simulink model "feedbackLin_Sim_Model"  (R2021a)
settings: Solver=ode1  StartTime=0.0  StopTime=200  FixedStep=0.005  RelTol=1e-3
values from neighbouring files (symbols this model uses):
  g = 9.31    [Metrics_Info.m]    (also in initEnv.m)
undefined symbols (not defined in the file or in its folder): Controller, DiscIntNeverNeededParam, Earth, init, rho, Vehicle, WGS84
libraries: shared6dof x1, aerolibasang x1, dynamicsLibrary x1, aerolibtransform2 x1
settings Model: Creator=laberobotica  LastModifiedBy=laberobotica

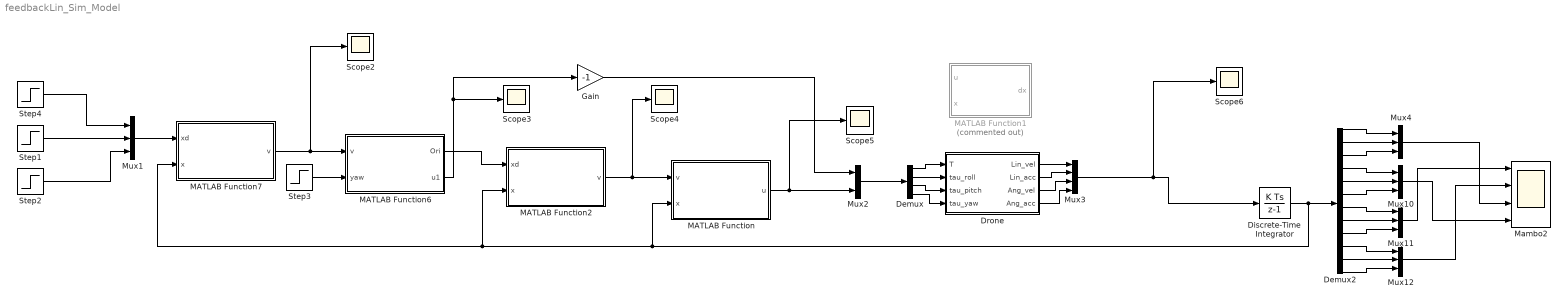
== system feedbackLin_Sim_Model ==
  Demux : Demux
  Demux2 : Demux  Outputs=12
  Discrete-Time Integrator : DiscreteIntegrator  SampleTime=0.005  ICPrevOutput=DiscIntNeverNeededParam  ICPrevScaledInput=DiscIntNeverNeededParam
  Drone : Subsystem
  Gain : Gain  Gain=-1
  MATLAB Function : MATLAB Function  TreatAsAtomicUnit=on
  MATLAB Function1 : MATLAB Function  Commented=on  TreatAsAtomicUnit=on
  MATLAB Function2 : MATLAB Function  TreatAsAtomicUnit=on
  MATLAB Function6 : MATLAB Function  TreatAsAtomicUnit=on
  MATLAB Function7 : MATLAB Function  TreatAsAtomicUnit=on
  Mambo2 : Scope  NumInputPorts=4
  Mux{1,4,10..12} (5 alike) : Mux  Inputs=3
  Mux2 : Mux  Inputs=2
  Mux3 : Mux
  Scope{2..6} (5 alike) : Scope
  Step1 : Step  Time=30  SampleTime=0
  Step2 : Step  Time=5  SampleTime=0.005
  Step3 : Step  Time=100  SampleTime=0.005
  Step4 : Step  Time=50  SampleTime=0
  wires:
  MATLAB Function2/1(v) -> Scope4/1, MATLAB Function/1(v)
  Mux1/1 -> MATLAB Function7/1(xd)
  Step2/1 -> Mux1/3
  MATLAB Function7/1(v) -> Scope2/1, MATLAB Function6/1(v)
  Demux2/7 -> Mux11/1
  Demux2/9 -> Mux11/3
  Demux2/2 -> Mux4/2
  Demux2/10 -> Mux12/1
  Mux11/1 -> Mambo2/1
  Mux4/1 -> Mambo2/3
  Demux2/8 -> Mux11/2
  Discrete-Time Integrator/1 -> MATLAB Function2/2(x), MATLAB Function7/2(x), MATLAB Function/2(x), Demux2/1
  Mux10/1 -> Mambo2/4
  Mux12/1 -> Mambo2/2
  Demux2/3 -> Mux4/3
  Demux2/11 -> Mux12/2
  Demux2/6 -> Mux10/3
  Demux2/12 -> Mux12/3
  Demux2/4 -> Mux10/1
  Demux2/5 -> Mux10/2
  Demux2/1 -> Mux4/1
  MATLAB Function6/2(u1) -> Gain/1, Scope3/1
  MATLAB Function6/1(Ori) -> MATLAB Function2/1(xd)
  Step4/1 -> Mux1/1
  Step1/1 -> Mux1/2
  Step3/1 -> MATLAB Function6/2(yaw)
  Drone/1(Lin_vel) -> Mux3/1
  Drone/2(Lin_acc) -> Mux3/2
  Drone/3(Ang_vel) -> Mux3/3
  Drone/4(Ang_acc) -> Mux3/4
  Demux/1 -> Drone/1(T)
  Demux/2 -> Drone/2(tau_roll)
  Demux/3 -> Drone/3(tau_pitch)
  Demux/4 -> Drone/4(tau_yaw)
  Mux3/1 -> Scope6/1, Discrete-Time Integrator/1
  Mux2/1 -> Demux/1
  Gain/1 -> Mux2/1
  MATLAB Function/1(u) -> Mux2/2, Scope5/1

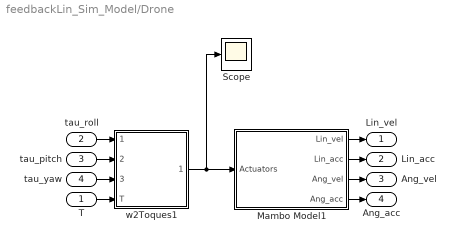
== system feedbackLin_Sim_Model/Drone ==
  T : Inport
  tau_roll : Inport  Port=2
  tau_pitch : Inport  Port=3
  tau_yaw : Inport  Port=4
  Mambo Model1 : Subsystem
  Scope : Scope
  w2Toques1 : Subsystem
  Lin_vel : Outport
  Lin_acc : Outport  Port=2
  Ang_vel : Outport  Port=3
  Ang_acc : Outport  Port=4
  wires:
  tau_yaw/1 -> w2Toques1/3(tau_yaw)
  tau_pitch/1 -> w2Toques1/2(tau_pitch)
  Mambo Model1/1(Lin_vel) -> Lin_vel/1
  Mambo Model1/4(Ang_acc) -> Ang_acc/1
  w2Toques1/1(Motors) -> Scope/1, Mambo Model1/1(Actuators)
  T/1 -> w2Toques1/4(T)
  Mambo Model1/3(Ang_vel) -> Ang_vel/1
  tau_roll/1 -> w2Toques1/1(tau_roll)
  Mambo Model1/2(Lin_acc) -> Lin_acc/1

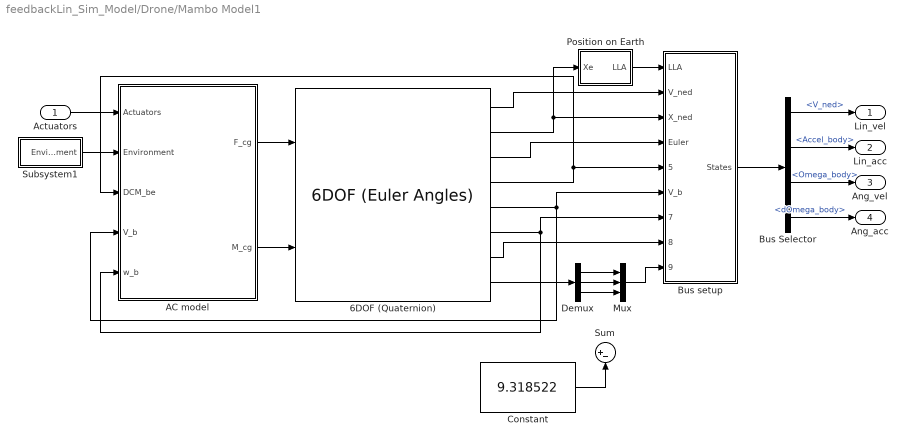
== system feedbackLin_Sim_Model/Drone/Mambo Model1 ==
  Actuators : Inport
  6DOF (Quaternion) : shared6dof/6DOF (Euler Angles)  units=Metric (MKS)  mtype=Fixed  rep=Euler Angles  xme_0=[0 0 0]  Vm_0=init.vb  eul_0=init.euler  pm_0=init.angRates  mass_0=Vehicle.Airframe.mass  mass_e=0.5  mass_f=2.0  inertia=Vehicle.Airframe.inertia  inertia_e=eye(3)  inertia_f=2*eye(3)  k_quat=Vehicle.SixDOF.quatGain  vre_flag=on  abi_flag=off  aMode=aMode  xme_statename=''  Vm_statename=''  eul_statename=''  quat_statename=''  pm_statename=''  mass_statename=''
      settings: SourceProductBaseCode=AE,PW,DR,MT,UV,VE
  AC model : Subsystem
  Bus Selector : BusSelector  OutputSignals=V_ned,Accel_body,Omega_body,dOmega_body
  Bus setup : Subsystem
  Constant : Constant  Value=9.318522
  Demux : Demux  Outputs=3
  Mux : Mux  Inputs=3
  Position on Earth : Subsystem  Priority=1  TreatAsAtomicUnit=on
  Subsystem1 : Subsystem
  Sum : Sum  Inputs=|+-
  Lin_vel : Outport
  Lin_acc : Outport  Port=2
  Ang_vel : Outport  Port=3
  Ang_acc : Outport  Port=4
  wires:
  Position on Earth/1(LLA) -> Bus setup/1(LLA)
  6DOF (Quaternion)/5 -> Bus setup/6(V_b), AC model/4(V_b)
  6DOF (Quaternion)/7 -> Bus setup/8(dOmega_b)
  Subsystem1/1(Environment) -> AC model/2(Environment)
  6DOF (Quaternion)/1 -> Bus setup/2(V_ned)
  Bus setup/1(States) -> Bus Selector/1
  AC model/1(F_cg) -> 6DOF (Quaternion)/1
  6DOF (Quaternion)/6 -> Bus setup/7(Omega_b), AC model/5(w_b)
  6DOF (Quaternion)/2 -> Position on Earth/1(Xe), Bus setup/3(X_ned)
  6DOF (Quaternion)/3 -> Bus setup/4(Euler)
  Actuators/1 -> AC model/1(Actuators)
  AC model/2(M_cg) -> 6DOF (Quaternion)/2
  6DOF (Quaternion)/4 -> AC model/3(DCM_be), Bus setup/5(DCM_be)
  Bus Selector/1 -> Lin_vel/1  "<V_ned>"
  Bus Selector/2 -> Lin_acc/1  "<Accel_body>"
  Bus Selector/3 -> Ang_vel/1  "<Omega_body>"
  Bus Selector/4 -> Ang_acc/1  "<dOmega_body>"
  Constant/1 -> Sum/2
  6DOF (Quaternion)/8 -> Demux/1
  Mux/1 -> Bus setup/9(Accel_b)
  Demux/1 -> Mux/1
  Demux/2 -> Mux/2
  Demux/3 -> Mux/3

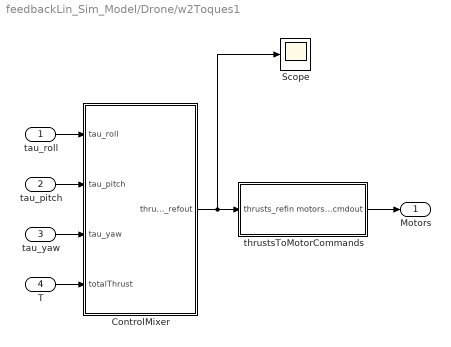
== system feedbackLin_Sim_Model/Drone/w2Toques1 ==
  tau_roll : Inport
  tau_pitch : Inport  Port=2
  tau_yaw : Inport  Port=3
  T : Inport  Port=4
  ControlMixer : Subsystem
  Scope : Scope
  thrustsToMotorCommands : Subsystem
  Motors : Outport  VectorParamsAs1DForOutWhenUnconnected=off
  wires:
  ControlMixer/1(thrusts_refout) -> Scope/1, thrustsToMotorCommands/1(thrusts_refin)
  thrustsToMotorCommands/1(motors_cmdout) -> Motors/1
  tau_roll/1 -> ControlMixer/1(tau_roll)
  tau_pitch/1 -> ControlMixer/2(tau_pitch)
  tau_yaw/1 -> ControlMixer/3(tau_yaw)
  T/1 -> ControlMixer/4(totalThrust)

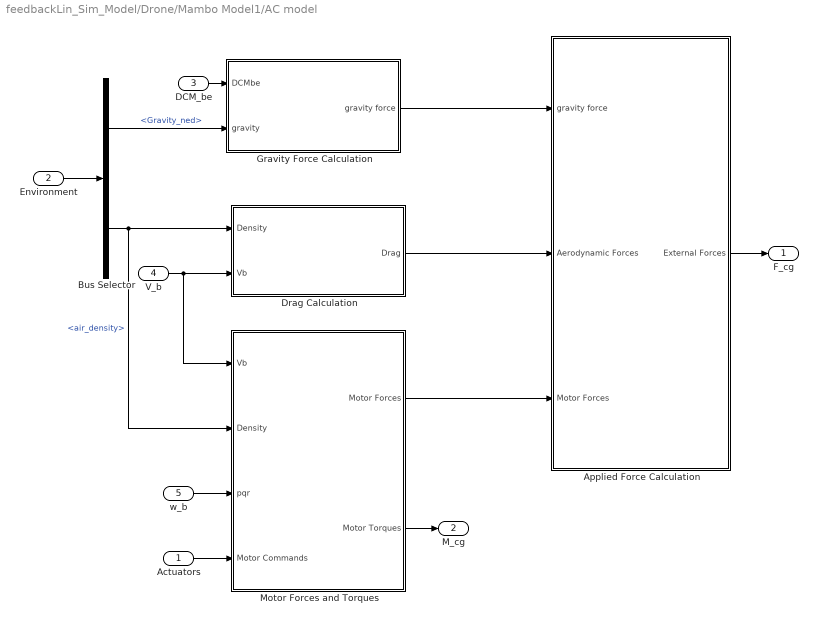
== system feedbackLin_Sim_Model/Drone/Mambo Model1/AC model ==
  Actuators : Inport
  Environment : Inport  Port=2
  DCM_be : Inport  Port=3
  V_b : Inport  Port=4  Unit=m/s
  w_b : Inport  Port=5  Unit=rad/s
  Applied Force Calculation : Subsystem
  Bus Selector : BusSelector  OutputSignals=Gravity_ned,AtmosphereBus.air_density
  Drag Calculation : Subsystem
  Gravity Force Calculation : Subsystem
  Motor Forces and Torques : Subsystem
  F_cg : Outport  Unit=N  VectorParamsAs1DForOutWhenUnconnected=off
  M_cg : Outport  Port=2  Unit=N*m  VectorParamsAs1DForOutWhenUnconnected=off
  wires:
  Bus Selector/1 -> Gravity Force Calculation/2(gravity)  "<Gravity_ned>"
  Gravity Force Calculation/1(gravity force) -> Applied Force Calculation/1(gravity force)
  Environment/1 -> Bus Selector/1
  Bus Selector/2 -> Motor Forces and Torques/2(Density), Drag Calculation/1(Density)  "<air_density>"
  DCM_be/1 -> Gravity Force Calculation/1(DCMbe)
  V_b/1 -> Motor Forces and Torques/1(Vb), Drag Calculation/2(Vb)
  Drag Calculation/1(Drag) -> Applied Force Calculation/2(Aerodynamic Forces)
  Actuators/1 -> Motor Forces and Torques/4(Motor Commands)
  w_b/1 -> Motor Forces and Torques/3(pqr)
  Motor Forces and Torques/2(Motor Torques) -> M_cg/1
  Applied Force Calculation/1(External Forces) -> F_cg/1
  Motor Forces and Torques/1(Motor Forces) -> Applied Force Calculation/3(Motor Forces)

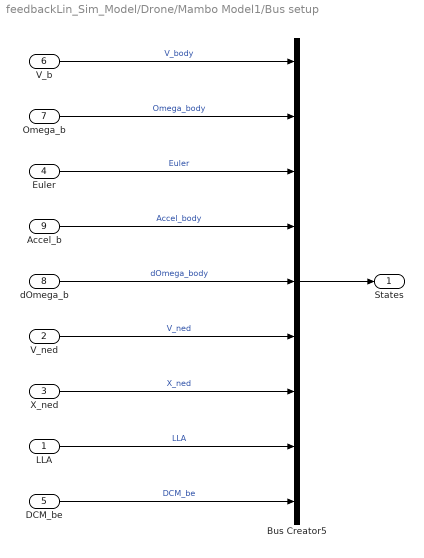
== system feedbackLin_Sim_Model/Drone/Mambo Model1/Bus setup ==
  LLA : Inport  PortDimensions=3
  V_ned : Inport  Port=2  Unit=m/second  PortDimensions=3
  X_ned : Inport  Port=3  Unit=m  PortDimensions=3
  Euler : Inport  Port=4  Unit=rad  PortDimensions=3
  DCM_be : Inport  Port=5  PortDimensions=[3 3]
  V_b : Inport  Port=6  Unit=m/s  PortDimensions=3
  Omega_b : Inport  Port=7  Unit=rad/s  PortDimensions=3
  dOmega_b : Inport  Port=8  Unit=rad/s^2  PortDimensions=3
  Accel_b : Inport  Port=9  Unit=m/s^2  PortDimensions=3
  Bus Creator5 : BusCreator  Inputs=9  OutDataTypeStr=Bus: StatesBus  NonVirtualBus=on
  States : Outport  VectorParamsAs1DForOutWhenUnconnected=off
  wires:
  Bus Creator5/1 -> States/1
  V_b/1 -> Bus Creator5/1  "V_body"
  Omega_b/1 -> Bus Creator5/2  "Omega_body"
  Euler/1 -> Bus Creator5/3  "Euler"
  X_ned/1 -> Bus Creator5/7  "X_ned"
  Accel_b/1 -> Bus Creator5/4  "Accel_body"
  LLA/1 -> Bus Creator5/8  "LLA"
  dOmega_b/1 -> Bus Creator5/5  "dOmega_body"
  DCM_be/1 -> Bus Creator5/9  "DCM_be"
  V_ned/1 -> Bus Creator5/6  "V_ned"

== system feedbackLin_Sim_Model/Drone/Mambo Model1/Position on Earth ==
  Xe : Inport  Unit=m
  Flat Earth to LLA : aerolibtransform2/Flat Earth to LLA  units=Metric (MKS)  ptype=Earth (WGS84)  F=1/298.257223563  R=6378137  refPosPort=off  LL0=init.posLLA(1:2)  psi=Vehicle.PositionOnEarth.FlatEarthToLLA.xAxis
  Mux : Mux  Inputs=2
  href : Constant  Value=Vehicle.PositionOnEarth.href
  LLA : Outport  VectorParamsAs1DForOutWhenUnconnected=off
  wires:
  Mux/1 -> LLA/1
  Xe/1 -> Flat Earth to LLA/1
  Flat Earth to LLA/1 -> Mux/1
  Flat Earth to LLA/2 -> Mux/2
  href/1 -> Flat Earth to LLA/2

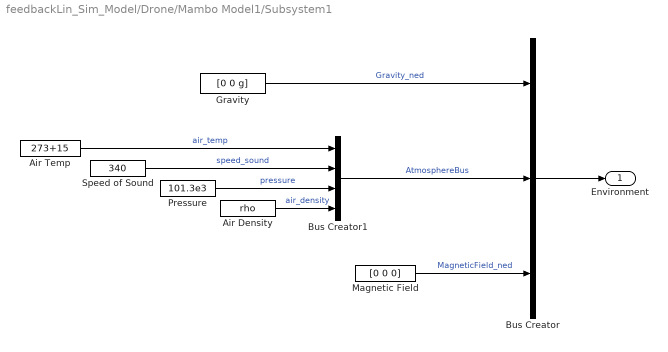
== system feedbackLin_Sim_Model/Drone/Mambo Model1/Subsystem1 ==
  Air Density : Constant  Value=rho
  Air Temp : Constant  Value=273+15
  Bus Creator : BusCreator  Inputs=3  OutDataTypeStr=Bus: EnvironmentBus  NonVirtualBus=on
  Bus Creator1 : BusCreator  Inputs=4  OutDataTypeStr=Bus: AtmosphereBus  NonVirtualBus=on
  Gravity : Constant  Value=[0 0 g]
  Magnetic Field : Constant  Value=[0 0 0]
  Pressure : Constant  Value=101.3e3
  Speed of Sound : Constant  Value=340
  Environment : Outport  VectorParamsAs1DForOutWhenUnconnected=off
  wires:
  Bus Creator1/1 -> Bus Creator/2  "AtmosphereBus"
  Gravity/1 -> Bus Creator/1  "Gravity_ned"
  Air Density/1 -> Bus Creator1/4  "air_density"
  Air Temp/1 -> Bus Creator1/1  "air_temp"
  Speed of Sound/1 -> Bus Creator1/2  "speed_sound"
  Magnetic Field/1 -> Bus Creator/3  "MagneticField_ned"
  Bus Creator/1 -> Environment/1
  Pressure/1 -> Bus Creator1/3  "pressure"

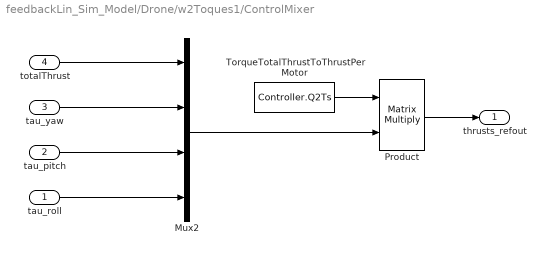
== system feedbackLin_Sim_Model/Drone/w2Toques1/ControlMixer ==
  tau_roll : Inport
  tau_pitch : Inport  Port=2
  tau_yaw : Inport  Port=3
  totalThrust : Inport  Port=4
  Mux2 : Mux
  Product : Product  Multiplication=Matrix(*)  RndMeth=Zero
  TorqueTotalThrustToThrustPerMotor : Constant  Value=Controller.Q2Ts  OutDataTypeStr=single
  thrusts_refout : Outport  VectorParamsAs1DForOutWhenUnconnected=off
  wires:
  Product/1 -> thrusts_refout/1
  tau_roll/1 -> Mux2/4
  tau_yaw/1 -> Mux2/2
  totalThrust/1 -> Mux2/1
  TorqueTotalThrustToThrustPerMotor/1 -> Product/1
  Mux2/1 -> Product/2
  tau_pitch/1 -> Mux2/3

== system feedbackLin_Sim_Model/Drone/w2Toques1/thrustsToMotorCommands ==
  thrusts_refin : Inport
  MotorDirections : Gain  Gain=[1 -1 1 -1]
  Saturation5 : Saturate  UpperLimit=Vehicle.Motor.maxLimit  LowerLimit=Vehicle.Motor.minLimit
  ThrustToMotorCommand : Gain  Gain=-Vehicle.Motor.thrustToMotorCommand
  motors_cmdout : Outport  VectorParamsAs1DForOutWhenUnconnected=off
  wires:
  Saturation5/1 -> MotorDirections/1
  MotorDirections/1 -> motors_cmdout/1
  ThrustToMotorCommand/1 -> Saturation5/1
  thrusts_refin/1 -> ThrustToMotorCommand/1

== system feedbackLin_Sim_Model/Drone/Mambo Model1/AC model/Applied Force Calculation ==
  gravity force : Inport  Unit=N
  Aerodynamic Forces : Inport  Port=2  Unit=N
  Motor Forces : Inport  Port=3  Unit=N
  Add1 : Sum  Inputs=+++
  Signal Specification : SignalSpecification  Dimensions=3
  External Forces : Outport  Unit=N  VectorParamsAs1DForOutWhenUnconnected=off
  wires:
  Add1/1 -> Signal Specification/1
  Motor Forces/1 -> Add1/3  "Motor Thrust"
  Aerodynamic Forces/1 -> Add1/2
  gravity force/1 -> Add1/1
  Signal Specification/1 -> External Forces/1

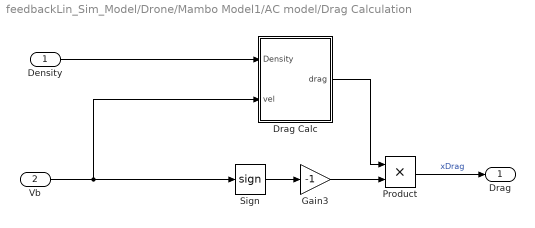
== system feedbackLin_Sim_Model/Drone/Mambo Model1/AC model/Drag Calculation ==
  Density : Inport  Unit=kg/m^3
  Vb : Inport  Port=2  Unit=m/second
  Drag Calc : Subsystem
  Gain3 : Gain  Gain=-1
  Product : Product  RndMeth=Zero
  Sign : Signum  ZeroCross=off
  Drag : Outport  Unit=N  VectorParamsAs1DForOutWhenUnconnected=off
  wires:
  Density/1 -> Drag Calc/1(Density)
  Sign/1 -> Gain3/1
  Drag Calc/1(drag) -> Product/1
  Gain3/1 -> Product/2
  Product/1 -> Drag/1  "xDrag"
  Vb/1 -> Sign/1, Drag Calc/2(vel)

== system feedbackLin_Sim_Model/Drone/Mambo Model1/AC model/Gravity Force Calculation ==
  DCMbe : Inport
  gravity : Inport  Port=2  Unit=m/s^2
  Gain1 : Gain  Gain=Vehicle.Airframe.mass
  Product : Product  Multiplication=Matrix(*)
  gravity force : Outport  Unit=N  VectorParamsAs1DForOutWhenUnconnected=off
  wires:
  gravity/1 -> Gain1/1
  Gain1/1 -> Product/2  "gravity force NED"
  Product/1 -> gravity force/1
  DCMbe/1 -> Product/1

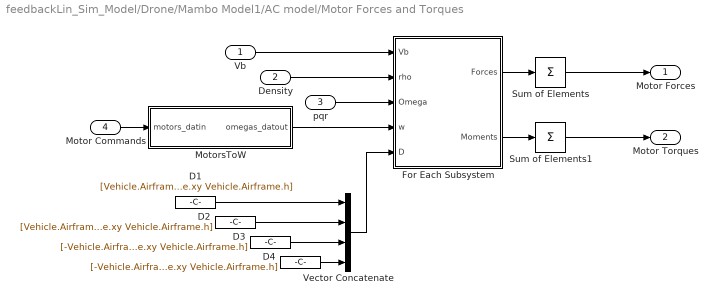
== system feedbackLin_Sim_Model/Drone/Mambo Model1/AC model/Motor Forces and Torques ==
  Vb : Inport
  Density : Inport  Port=2
  pqr : Inport  Port=3
  Motor Commands : Inport  Port=4
  D1 : Constant  Value=[Vehicle.Airframe.xy -Vehicle.Airframe.xy Vehicle.Airframe.h]
  D2 : Constant  Value=[Vehicle.Airframe.xy Vehicle.Airframe.xy Vehicle.Airframe.h]
  D3 : Constant  Value=[-Vehicle.Airframe.xy Vehicle.Airframe.xy Vehicle.Airframe.h]
  D4 : Constant  Value=[-Vehicle.Airframe.xy -Vehicle.Airframe.xy Vehicle.Airframe.h]
  For Each Subsystem : Subsystem  TreatAsAtomicUnit=on
  MotorsToW : Subsystem
  Sum of Elements : Sum  Inputs=+  CollapseMode=Specified dimension  CollapseDim=2
  Sum of Elements1 : Sum  Inputs=+  CollapseMode=Specified dimension  CollapseDim=2
  Vector Concatenate : Concatenate  NumInputs=4  Mode=Multidimensional array  ConcatenateDimension=2
  Motor Forces : Outport  Unit=N  VectorParamsAs1DForOutWhenUnconnected=off
  Motor Torques : Outport  Port=2  Unit=N*m  VectorParamsAs1DForOutWhenUnconnected=off
  wires:
  D4/1 -> Vector Concatenate/4
  MotorsToW/1(omegas_datout) -> For Each Subsystem/4(w)
  Vector Concatenate/1 -> For Each Subsystem/5(D)
  For Each Subsystem/2(Moments) -> Sum of Elements1/1
  pqr/1 -> For Each Subsystem/3(Omega)
  Vb/1 -> For Each Subsystem/1(Vb)
  Motor Commands/1 -> MotorsToW/1(motors_datin)
  D1/1 -> Vector Concatenate/1
  D3/1 -> Vector Concatenate/3
  D2/1 -> Vector Concatenate/2
  Sum of Elements1/1 -> Motor Torques/1
  Density/1 -> For Each Subsystem/2(rho)
  Sum of Elements/1 -> Motor Forces/1
  For Each Subsystem/1(Forces) -> Sum of Elements/1

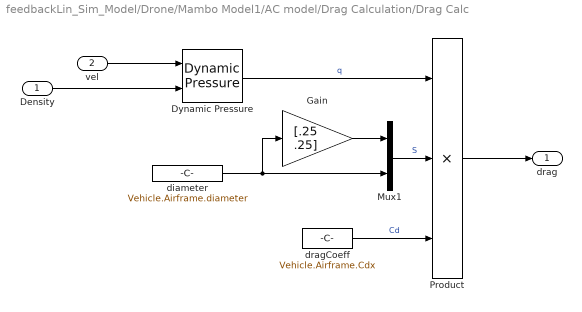
== system feedbackLin_Sim_Model/Drone/Mambo Model1/AC model/Drag Calculation/Drag Calc ==
  Density : Inport  Unit=kg/m^3
  vel : Inport  Port=2  Unit=m/s
  Dynamic Pressure : aerolibasang/Dynamic Pressure
  Gain : Gain  Gain=[.25 .25]
  Mux1 : Mux  Inputs=2
  Product : Product  Inputs=3  RndMeth=Zero
  diameter : Constant  Value=Vehicle.Airframe.diameter  SampleTime=0
  dragCoeff : Constant  Value=Vehicle.Airframe.Cdx  SampleTime=0
  drag : Outport  Unit=N  VectorParamsAs1DForOutWhenUnconnected=off
  wires:
  Product/1 -> drag/1
  dragCoeff/1 -> Product/3  "Cd"
  Dynamic Pressure/1 -> Product/1  "q"
  diameter/1 -> Gain/1, Mux1/2
  Mux1/1 -> Product/2  "S"
  Gain/1 -> Mux1/1
  vel/1 -> Dynamic Pressure/1
  Density/1 -> Dynamic Pressure/2

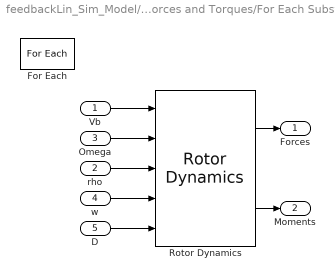
== system feedbackLin_Sim_Model/Drone/Mambo Model1/AC model/Motor Forces and Torques/For Each Subsystem ==
  Vb : Inport  PortDimensions=3
  rho : Inport  Port=2  PortDimensions=1
  Omega : Inport  Port=3
  w : Inport  Port=4  Partition=on  PartitionDimension=1  PartitionWidth=1  PartitionOffset=0
  D : Inport  Port=5  Partition=on  PartitionDimension=2  PartitionWidth=1  PartitionOffset=0
  For Each : ForEach  DisableCoverage=on
  Rotor Dynamics : dynamicsLibrary/Rotor Dynamics  SystemSampleTime=-1  VariantActivationTime=update diagram  Latency=0  AutoFrameSizeCalculation=off
  Forces : Outport  ConcatenationDimension=2  VectorParamsAs1DForOutWhenUnconnected=off
  Moments : Outport  Port=2  ConcatenationDimension=2  VectorParamsAs1DForOutWhenUnconnected=off
  wires:
  Rotor Dynamics/1 -> Forces/1
  Rotor Dynamics/2 -> Moments/1
  Vb/1 -> Rotor Dynamics/1
  Omega/1 -> Rotor Dynamics/2
  rho/1 -> Rotor Dynamics/3
  D/1 -> Rotor Dynamics/5
  w/1 -> Rotor Dynamics/4

== system feedbackLin_Sim_Model/Drone/Mambo Model1/AC model/Motor Forces and Torques/MotorsToW ==
  motors_datin : Inport
  Motordirections : Gain  Gain=[1 -1 1 -1]  ParamDataTypeStr=single  OutDataTypeStr=Inherit: Inherit via back propagation  SaturateOnIntegerOverflow=on
  Motordirections1 : Gain  Gain=[1 -1 1 -1]  ParamDataTypeStr=single  OutDataTypeStr=Inherit: Inherit via back propagation  SaturateOnIntegerOverflow=on
  Saturation5 : Saturate  UpperLimit=Vehicle.Motor.maxLimit  LowerLimit=Vehicle.Motor.minLimit  OutDataTypeStr=Inherit: Inherit via back propagation
  Signed Sqrt : Sqrt  Operator=signedSqrt  OutDataTypeStr=Inherit: Inherit via back propagation  SaturateOnIntegerOverflow=on
  motorsToW2_Gain : Gain  Gain=Vehicle.Motor.commandToW2Gain  ParamDataTypeStr=single  OutDataTypeStr=Inherit: Inherit via back propagation  SaturateOnIntegerOverflow=on
  omegas_datout : Outport  VectorParamsAs1DForOutWhenUnconnected=off
  wires:
  motorsToW2_Gain/1 -> Signed Sqrt/1
  Motordirections/1 -> Saturation5/1
  Saturation5/1 -> Motordirections1/1
  Motordirections1/1 -> motorsToW2_Gain/1
  Signed Sqrt/1 -> omegas_datout/1
  motors_datin/1 -> Motordirections/1

== matlab function feedbackLin_Sim_Model/MATLAB Function1 ==
  data: u input; dx output; x input
function dx  = DroneModel(u,x)

g = 9.81;
m = 0.063;
l = 0.0624*2;
Jx = 5.82857e-5;
Jy = 7.169148e-5;
Jz = 1e-4;

dx = zeros(1,12);

dx(1) = x(4);
dx(2) = x(5);
dx(3) = x(6);

dx(4) = -(cos(x(7)) * sin(x(8)) * cos(x(9)) + sin(x(7))*sin(x(9)))*(u(1)/m);

dx(5) = -(cos(x(7)) * sin(x(8)) * sin(x(9)) - sin(x(7))*cos(x(9)))*(u(1)/m);

dx(6) = g- (cos(x(7)) * cos(x(8)))*(u(1)/m);

dx(7) = x(10);
dx(8) = x(11);
dx(9) = x(12);

dx(10) = x(11)*x(12)*((Jy-Jz)/Jx)+(l/Jx)*u(2);
dx(11) = x(10)*x(12)*((Jz-Jx)/Jy)+(l/Jy)*u(3);
dx(12) = x(10)*x(11)*((Jx-Jy)/Jz)+(1/Jz)*u(4);
end

== matlab function feedbackLin_Sim_Model/MATLAB Function ==
  data: v input; u output; x input
function u = feedBackLinAtt(v, x)
g = 9.31;

m = 0.063;
l = 0.0624*2;
Jx = 5.82857e-5;
Jy = 7.169148e-5;
Jz = 1e-4;
K4 = -8; K3 = -8; K2 = -8;

u = zeros(1,3);

u(1) = (Jx/l)*(K2*x(10)-x(11)*x(12)*((Jy-Jz)/Jx))+v(1);
u(2) = (Jy/l)*(K3*x(11)-x(10)*x(12)*((Jz-Jx)/Jy))+v(2);
u(3) = (Jz)*(K4*x(12)-x(10)*x(11)*((Jx-Jy)/Jz))+v(3);
end

== matlab function feedbackLin_Sim_Model/MATLAB Function2 ==
  data: xd input; x input; v output
function v = ControlAttidude(xd,x)

w2 = 0.0075; w3 = 0.0075; w4 = 0.00075;
v = zeros(1,3);

% controle de orientação
v(1) = w2*(xd(1) - x(7));
v(2) = w3*(xd(2) - x(8));
v(3) = w4*(xd(3) - x(9));


end

== matlab function feedbackLin_Sim_Model/MATLAB Function6 ==
  data: v input; Ori output; u1 output; yaw input
function [Ori,u1] = feedBackLinAlt(v,yaw)
g = 9.81;
m = 0.063;
l = 0.0624*2;
Jx = 5.82857e-5;
Jy = 7.169148e-5;
Jz = 1e-4;
Ori = zeros(1,3);
u1=0;

u1 = m*((v(1)^2)+(v(2)^2)+((g-v(3))^2))^0.5;  %m*sqrt(((v(1)/beta)^2)+v(2)^2)

beta = (v(1)/u1)*m;

alpha = (v(2)/u1)*m;

Ori(1)=asin(alpha);
Ori(2)=-asin(beta);
Ori(3) = yaw;


end

== matlab function feedbackLin_Sim_Model/MATLAB Function7 ==
  data: xd input; x input; v output
function v = ControlAlt(xd,x)

k1 = 0.1; k2=0.1; k3=0.1;
v = zeros(1,3);


v(1) = k1*(xd(1) - x(1))+(-0.5*x(4));%
v(2) = k2*(xd(2) - x(2))+(-0.5*x(5));
v(3) = k3*(xd(3) - x(3))+(-0.5*x(6));

end
